simulink model "three_phase_pwm_rectifier_ac_dc_conv_simscape"  (R2019a)
settings: Solver=ode23t  StartTime=0.0  StopTime=2  MaxStep=1e-6  RelTol=1e-6
values from neighbouring files (symbols this model uses):
  Co = 10e-3    (= 0.01)    [design_parameters.m]
  fline = 50    [design_parameters.m]
  K = (3/2)*(Vm/Vdc)    (= 0.609375)    [design_parameters.m]
  Kic = Kpc/Tc    (= 4545.45454545)    [design_parameters.m]
  Kipll = Kpll/Tpll    [design_parameters.m]
  Kiv = Kpv/Tv    [design_parameters.m]
  Kpc = Kc    (= 90.9090909091)    [design_parameters.m]
  Kpll = (1/Vm)*(1/(alfa_pll*Tsamp))    [design_parameters.m]
  Kpv = Kv    [design_parameters.m]
  Ls = 10e-3    (= 0.01)    [design_parameters.m]
  Rload = 200    [design_parameters.m]
  Rs = 0.5    [design_parameters.m]
  T1 = Tsamp/10    (= 5e-06)    [design_parameters.m]
  T2 = Tsamp/10    (= 5e-06)    [design_parameters.m]
  Tsamp = Tsw/2    (= 5e-05)    [design_parameters.m]
  Vdc = 800    [design_parameters.m]
  Vm = 325    [design_parameters.m]
undefined symbols (not defined in the file or in its folder): Iqe_max
libraries: powerlib x32, simulink x4, powerlib_meascontrol x1
settings Model: Creator=Görkem  LastModifiedBy=gsahi
settings DataIOCC: ReturnWorkspaceOutputs=off
settings DebuggingCC: ParameterOverflowMsg=none

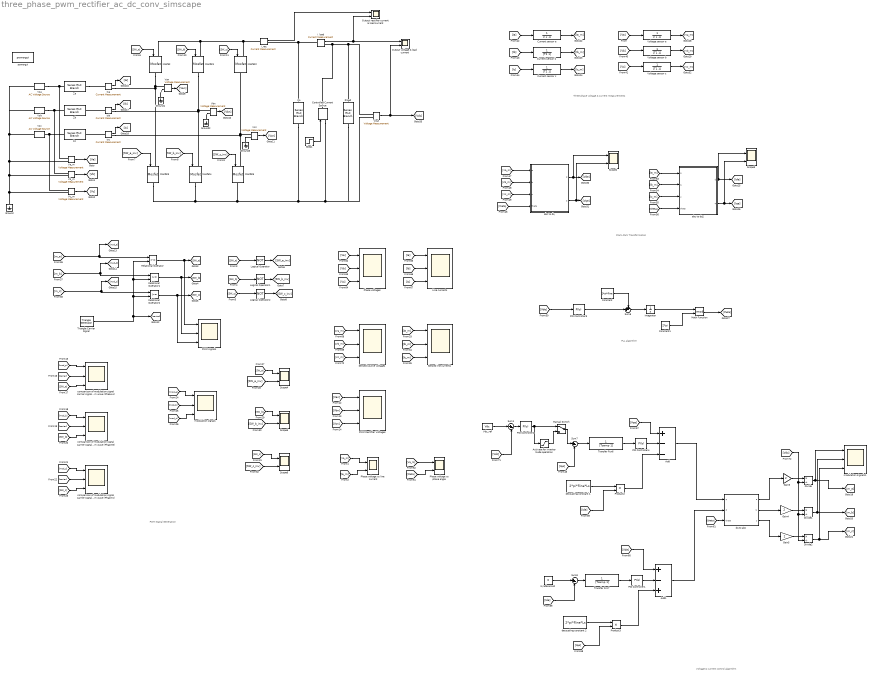
== system three_phase_pwm_rectifier_ac_dc_conv_simscape ==
  note: PWM Signal Generation
  note: Three phase voltage & current measurements
  note: Clark-Park Transformation
  note: PLL algorithm
  note: Voltage & current control algorithm
  "Activate for inverter mode operation " : Saturate  UpperLimit=-(Vdc/Rload)/K  LowerLimit=-20
  Add : Sum  Inputs=+--
  Add1 : Sum  Inputs=+-+
  Co : powerlib/Elements/Series RLC Branch  LConnTagsString=__new0  RConnTagsString=__new0  BranchType=C  Resistance=5  Inductance=1e-3  SetiL0=off  InitialCurrent=0  Capacitance=Co  Setx0=on  InitialVoltage=Vdc  Measurements=None
      settings: SourceProductName=Simscape Electrical
  Constant : Constant  Value=2*pi*fline
  Constant1 : Constant  Value=2*pi
  Controlled Current Source : powerlib/Electrical Sources/Controlled Current Source  Initialize=on  Source_Type=AC  Amplitude=0  Phase=0  Frequency=0  Measurements=None
      settings: SourceProductName=Simscape Electrical
  Current sensor a : TransferFcn  Denominator=[T2 1]
  Current sensor b : TransferFcn  Denominator=[T2 1]
  Current sensor c : TransferFcn  Denominator=[T2 1]
  Divide : Product  Inputs=*/
  Divide1 : Product  Inputs=*/
  Divide2 : Product  Inputs=*/
  Gain3 : Gain  Gain=2
  Gain4 : Gain  Gain=2
  Gain5 : Gain  Gain=2
  Ground{,1..3} (4 alike) : powerlib/Elements/Ground  LConnTagsString=a
      settings: SourceProductName=Simscape Electrical
  I_rec : powerlib/Measurements/Current Measurement  PhasorSimulation=off  OutputType=Complex  PSBequivalent=0
      settings: SourceProductName=Simscape Electrical
  Integrator : Integrator
  Iq reference2 : Constant  Value=0
  Isa : powerlib/Measurements/Current Measurement  PhasorSimulation=off  OutputType=Complex  PSBequivalent=0
      settings: SourceProductName=Simscape Electrical
  Isb : powerlib/Measurements/Current Measurement  PhasorSimulation=off  OutputType=Complex  PSBequivalent=0
      settings: SourceProductName=Simscape Electrical
  Isc : powerlib/Measurements/Current Measurement  PhasorSimulation=off  OutputType=Complex  PSBequivalent=0
      settings: SourceProductName=Simscape Electrical
  Line currents : Scope  NumInputPorts=3
  Logical Operator : Logic  Operator=NOT  AllPortsSameDT=off  OutDataTypeStr=boolean
  Logical Operator1 : Logic  Operator=NOT  AllPortsSameDT=off  OutDataTypeStr=boolean
  Logical Operator2 : Logic  Operator=NOT  AllPortsSameDT=off  OutDataTypeStr=boolean
  Manual Switch : ManualSwitch
  Math Function : Math  Operator=mod  SaturateOnIntegerOverflow=on
  Mosfet{,1..5} (6 alike) : powerlib/Power Electronics/Mosfet  Ron=0.1  Lon=0  Rd=0.01  Vfd=0  IC=0  Rs=1e5  Cs=inf  Measurements=off
      settings: SourceProductName=Simscape Electrical
  Output rectifier current & load current : Scope  NumInputPorts=2
  Output voltage & load current : Scope  NumInputPorts=2
  PID Controller1 : simulink/Continuous/PID Controller  Controller=PI  Form=Parallel  TimeDomain=Continuous-time  SampleTime=-1  IntegratorMethod=Forward Euler  FilterMethod=Forward Euler  ControllerParametersSource=internal  P=Kpc  I=Kic  D=0  UseFilter=on  N=100  TunerSelectOption=Transfer Function Based (PID Tuner App)  InitialConditionSource=internal  InitialConditionForIntegrator=0  InitialConditionForFilter=0  DifferentiatorICPrevScaledInput=0  ExternalReset=none  TrackingMode=off  Kt=1  LimitOutput=on  UpperSaturationLimit=400  LowerSaturationLimit=-400  LinearizeAsGain=on  AntiWindupMode=clamping  Kb=1  POutMin=[]  POutMax=[]  IOutMin=[]  IOutMax=[]  DOutMin=[]  DOutMax=[]  NOutMin=[]  NOutMax=[]  SumOutMin=[]  SumOutMax=[]  SaturationOutMin=[]  SaturationOutMax=[]  PParamMin=[]  PParamMax=[]  IParamMin=[]  IParamMax=[]  DParamMin=[]  DParamMax=[]  NParamMin=[]  NParamMax=[]  KbParamMin=[]  KbParamMax=[]  KtParamMin=[]  KtParamMax=[]  KbOutMin=[]  KbOutMax=[]  KtOutMin=[]  KtOutMax=[]  IntegratorOutMin=[]  IntegratorOutMax=[]  FilterOutMin=[]  FilterOutMax=[]  SumI1OutMin=[]  SumI1OutMax=[]  SumI2OutMin=[]  SumI2OutMax=[]  SumI3OutMin=[]  SumI3OutMax=[]  SumI4OutMin=[]  SumI4OutMax=[]  SumDOutMin=[]  SumDOutMax=[]  DifferentiatorOutMin=[]  DifferentiatorOutMax=[]  FilterDiffOutCoefMin=[]  FilterDiffOutCoefMax=[]  ReciprocalOutMin=[]  ReciprocalOutMax=[]  SumDenOutMin=[]  SumDenOutMax=[]  SumNumOutMin=[]  SumNumOutMax=[]  DivideOutMin=[]  DivideOutMax=[]  IntegratorContinuousStateAttributes=''  IntegratorStateMustResolveToSignalObject=off  IntegratorRTWStateStorageClass=Auto  FilterContinuousStateAttributes=''  FilterStateMustResolveToSignalObject=off  FilterRTWStateStorageClass=Auto  ParallelPVariant=InternalParameters  IdealPVariant=Disabled  IVariant=InternalParameters  DVariant=Disabled  IntegratorVariant=Continuous  SatVariant=Enabled  AWVariant=ContClampingParallel  PCopyVariant=Disabled  TRVariant=Disabled  FdbkBlocksVariant=Forward  IdealPFdbkVariant=Disabled  SatFdbkVariant=Disabled  DerivativeFilterVariant=Disabled  NVariant=Disabled  NCopyVariant=Disabled_SignalSpec  FilterICVariant=Disabled  IntegratorICVariant=InternalICs  ExternalResetVariant=Disabled  TRSumVariant=Passthrough  SumFdbkVariant=Disabled  SumVariant=Sum_PI
  PID Controller2 : simulink/Continuous/PID Controller  Controller=PI  Form=Parallel  TimeDomain=Continuous-time  SampleTime=-1  IntegratorMethod=Forward Euler  FilterMethod=Forward Euler  ControllerParametersSource=internal  P=Kpv  I=Kiv  D=0  UseFilter=on  N=100  TunerSelectOption=Transfer Function Based (PID Tuner App)  InitialConditionSource=internal  InitialConditionForIntegrator=0  InitialConditionForFilter=0  DifferentiatorICPrevScaledInput=0  ExternalReset=none  TrackingMode=off  Kt=1  LimitOutput=off  UpperSaturationLimit=Iqe_max  LowerSaturationLimit=-Iqe_max  LinearizeAsGain=on  AntiWindupMode=clamping  Kb=1  POutMin=[]  POutMax=[]  IOutMin=[]  IOutMax=[]  DOutMin=[]  DOutMax=[]  NOutMin=[]  NOutMax=[]  SumOutMin=[]  SumOutMax=[]  SaturationOutMin=[]  SaturationOutMax=[]  PParamMin=[]  PParamMax=[]  IParamMin=[]  IParamMax=[]  DParamMin=[]  DParamMax=[]  NParamMin=[]  NParamMax=[]  KbParamMin=[]  KbParamMax=[]  KtParamMin=[]  KtParamMax=[]  KbOutMin=[]  KbOutMax=[]  KtOutMin=[]  KtOutMax=[]  IntegratorOutMin=[]  IntegratorOutMax=[]  FilterOutMin=[]  FilterOutMax=[]  SumI1OutMin=[]  SumI1OutMax=[]  SumI2OutMin=[]  SumI2OutMax=[]  SumI3OutMin=[]  SumI3OutMax=[]  SumI4OutMin=[]  SumI4OutMax=[]  SumDOutMin=[]  SumDOutMax=[]  DifferentiatorOutMin=[]  DifferentiatorOutMax=[]  FilterDiffOutCoefMin=[]  FilterDiffOutCoefMax=[]  ReciprocalOutMin=[]  ReciprocalOutMax=[]  SumDenOutMin=[]  SumDenOutMax=[]  SumNumOutMin=[]  SumNumOutMax=[]  DivideOutMin=[]  DivideOutMax=[]  IntegratorContinuousStateAttributes=''  IntegratorStateMustResolveToSignalObject=off  IntegratorRTWStateStorageClass=Auto  FilterContinuousStateAttributes=''  FilterStateMustResolveToSignalObject=off  FilterRTWStateStorageClass=Auto  ParallelPVariant=InternalParameters  IdealPVariant=Disabled  IVariant=InternalParameters  DVariant=Disabled  IntegratorVariant=Continuous  SatVariant=Disabled  AWVariant=Passthrough  PCopyVariant=Disabled  TRVariant=Disabled  FdbkBlocksVariant=Forward  IdealPFdbkVariant=Disabled  SatFdbkVariant=Disabled  DerivativeFilterVariant=Disabled  NVariant=Disabled  NCopyVariant=Disabled_SignalSpec  FilterICVariant=Disabled  IntegratorICVariant=InternalICs  ExternalResetVariant=Disabled  TRSumVariant=Passthrough  SumFdbkVariant=Disabled  SumVariant=Sum_PI
  PID Controller3 : simulink/Continuous/PID Controller  Controller=PI  Form=Parallel  TimeDomain=Continuous-time  SampleTime=-1  IntegratorMethod=Forward Euler  FilterMethod=Forward Euler  ControllerParametersSource=internal  P=Kpll  I=Kipll  D=0  UseFilter=on  N=100  TunerSelectOption=Transfer Function Based (PID Tuner App)  InitialConditionSource=internal  InitialConditionForIntegrator=0  InitialConditionForFilter=0  DifferentiatorICPrevScaledInput=0  ExternalReset=none  TrackingMode=off  Kt=1  LimitOutput=off  UpperSaturationLimit=inf  LowerSaturationLimit=-inf  LinearizeAsGain=on  AntiWindupMode=none  Kb=1  POutMin=[]  POutMax=[]  IOutMin=[]  IOutMax=[]  DOutMin=[]  DOutMax=[]  NOutMin=[]  NOutMax=[]  SumOutMin=[]  SumOutMax=[]  SaturationOutMin=[]  SaturationOutMax=[]  PParamMin=[]  PParamMax=[]  IParamMin=[]  IParamMax=[]  DParamMin=[]  DParamMax=[]  NParamMin=[]  NParamMax=[]  KbParamMin=[]  KbParamMax=[]  KtParamMin=[]  KtParamMax=[]  KbOutMin=[]  KbOutMax=[]  KtOutMin=[]  KtOutMax=[]  IntegratorOutMin=[]  IntegratorOutMax=[]  FilterOutMin=[]  FilterOutMax=[]  SumI1OutMin=[]  SumI1OutMax=[]  SumI2OutMin=[]  SumI2OutMax=[]  SumI3OutMin=[]  SumI3OutMax=[]  SumI4OutMin=[]  SumI4OutMax=[]  SumDOutMin=[]  SumDOutMax=[]  DifferentiatorOutMin=[]  DifferentiatorOutMax=[]  FilterDiffOutCoefMin=[]  FilterDiffOutCoefMax=[]  ReciprocalOutMin=[]  ReciprocalOutMax=[]  SumDenOutMin=[]  SumDenOutMax=[]  SumNumOutMin=[]  SumNumOutMax=[]  DivideOutMin=[]  DivideOutMax=[]  IntegratorContinuousStateAttributes=''  IntegratorStateMustResolveToSignalObject=off  IntegratorRTWStateStorageClass=Auto  FilterContinuousStateAttributes=''  FilterStateMustResolveToSignalObject=off  FilterRTWStateStorageClass=Auto  ParallelPVariant=InternalParameters  IdealPVariant=Disabled  IVariant=InternalParameters  DVariant=Disabled  IntegratorVariant=Continuous  SatVariant=Disabled  AWVariant=Passthrough  PCopyVariant=Disabled  TRVariant=Disabled  FdbkBlocksVariant=Forward  IdealPFdbkVariant=Disabled  SatFdbkVariant=Disabled  DerivativeFilterVariant=Disabled  NVariant=Disabled  NCopyVariant=Disabled_SignalSpec  FilterICVariant=Disabled  IntegratorICVariant=InternalICs  ExternalResetVariant=Disabled  TRSumVariant=Passthrough  SumFdbkVariant=Disabled  SumVariant=Sum_PI
  PID Controller4 : simulink/Continuous/PID Controller  Controller=PI  Form=Parallel  TimeDomain=Continuous-time  SampleTime=-1  IntegratorMethod=Forward Euler  FilterMethod=Forward Euler  ControllerParametersSource=internal  P=Kpc  I=Kic  D=0  UseFilter=on  N=100  TunerSelectOption=Transfer Function Based (PID Tuner App)  InitialConditionSource=internal  InitialConditionForIntegrator=0  InitialConditionForFilter=0  DifferentiatorICPrevScaledInput=0  ExternalReset=none  TrackingMode=off  Kt=1  LimitOutput=on  UpperSaturationLimit=Vdc/2  LowerSaturationLimit=-Vdc/2  LinearizeAsGain=on  AntiWindupMode=clamping  Kb=1  POutMin=[]  POutMax=[]  IOutMin=[]  IOutMax=[]  DOutMin=[]  DOutMax=[]  NOutMin=[]  NOutMax=[]  SumOutMin=[]  SumOutMax=[]  SaturationOutMin=[]  SaturationOutMax=[]  PParamMin=[]  PParamMax=[]  IParamMin=[]  IParamMax=[]  DParamMin=[]  DParamMax=[]  NParamMin=[]  NParamMax=[]  KbParamMin=[]  KbParamMax=[]  KtParamMin=[]  KtParamMax=[]  KbOutMin=[]  KbOutMax=[]  KtOutMin=[]  KtOutMax=[]  IntegratorOutMin=[]  IntegratorOutMax=[]  FilterOutMin=[]  FilterOutMax=[]  SumI1OutMin=[]  SumI1OutMax=[]  SumI2OutMin=[]  SumI2OutMax=[]  SumI3OutMin=[]  SumI3OutMax=[]  SumI4OutMin=[]  SumI4OutMax=[]  SumDOutMin=[]  SumDOutMax=[]  DifferentiatorOutMin=[]  DifferentiatorOutMax=[]  FilterDiffOutCoefMin=[]  FilterDiffOutCoefMax=[]  ReciprocalOutMin=[]  ReciprocalOutMax=[]  SumDenOutMin=[]  SumDenOutMax=[]  SumNumOutMin=[]  SumNumOutMax=[]  DivideOutMin=[]  DivideOutMax=[]  IntegratorContinuousStateAttributes=''  IntegratorStateMustResolveToSignalObject=off  IntegratorRTWStateStorageClass=Auto  FilterContinuousStateAttributes=''  FilterStateMustResolveToSignalObject=off  FilterRTWStateStorageClass=Auto  ParallelPVariant=InternalParameters  IdealPVariant=Disabled  IVariant=InternalParameters  DVariant=Disabled  IntegratorVariant=Continuous  SatVariant=Enabled  AWVariant=ContClampingParallel  PCopyVariant=Disabled  TRVariant=Disabled  FdbkBlocksVariant=Forward  IdealPFdbkVariant=Disabled  SatFdbkVariant=Disabled  DerivativeFilterVariant=Disabled  NVariant=Disabled  NCopyVariant=Disabled_SignalSpec  FilterICVariant=Disabled  IntegratorICVariant=InternalICs  ExternalResetVariant=Disabled  TRSumVariant=Passthrough  SumFdbkVariant=Disabled  SumVariant=Sum_PI
  PWM Rectifier Voltages : Scope  NumInputPorts=3
  PWM signals : Scope  NumInputPorts=3
  Phase voltage vs line current : Scope  NumInputPorts=2
  Phase voltage vs phase angle : Scope  NumInputPorts=2
  Phase voltages : Scope  NumInputPorts=3
  Product2 : Product
  Product3 : Product
  Relational Operator : RelationalOperator  OutDataTypeStr=boolean  RndMeth=Simplest
  Relational Operator1 : RelationalOperator  OutDataTypeStr=boolean  RndMeth=Simplest
  Relational Operator2 : RelationalOperator  OutDataTypeStr=boolean  RndMeth=Simplest
  Rload : powerlib/Elements/Series RLC Branch  LConnTagsString=__new0  RConnTagsString=__new0  BranchType=R  Resistance=Rload  Inductance=1e-3  SetiL0=off  InitialCurrent=0  Capacitance=Co  Setx0=on  InitialVoltage=Vdc  Measurements=None
      settings: SourceProductName=Simscape Electrical
  Scope{2..6} (5 alike) : Scope  NumInputPorts=2
  Sensed line currents : Scope  NumInputPorts=3
  Sensed source voltages : Scope  NumInputPorts=3
  Step1 : Step  Time=0.05  After=-Vdc/(3*Rload)  SampleTime=0
  Sum1 : Sum  Inputs=|+-
  Sum6 : Sum  Inputs=++|
  Sum7 : Sum  Inputs=|+-
  Sum8 : Sum  Inputs=|+-
  Transfer Fcn6 : TransferFcn  Denominator=[Tsamp 1]
  Transfer Fcn7 : TransferFcn  Denominator=[Tsamp 1]
  Triangle Carrier Signal : powerlib_meascontrol/Pulse & Signal Generators/Triangle Generator  Freq=fsw  Phase=-90  Ts=0
      settings: SourceProductName=Simscape Electrical
  Va_m : powerlib/Measurements/Voltage Measurement  PhasorSimulation=off  OutputType=Complex  PSBequivalent=0
      settings: SourceProductName=Simscape Electrical
  Van : powerlib/Measurements/Voltage Measurement  PhasorSimulation=off  OutputType=Complex  PSBequivalent=0
      settings: SourceProductName=Simscape Electrical
  Vb_m : powerlib/Measurements/Voltage Measurement  PhasorSimulation=off  OutputType=Complex  PSBequivalent=0
      settings: SourceProductName=Simscape Electrical
  Vbn : powerlib/Measurements/Voltage Measurement  PhasorSimulation=off  OutputType=Complex  PSBequivalent=0
      settings: SourceProductName=Simscape Electrical
  Vc_m : powerlib/Measurements/Voltage Measurement  PhasorSimulation=off  OutputType=Complex  PSBequivalent=0
      settings: SourceProductName=Simscape Electrical
  Vcn : powerlib/Measurements/Voltage Measurement  PhasorSimulation=off  OutputType=Complex  PSBequivalent=0
      settings: SourceProductName=Simscape Electrical
  Vdc_ref : Constant  Value=Vdc
  Voltage sensor a : TransferFcn  Denominator=[T1 1]
  Voltage sensor b : TransferFcn  Denominator=[T1 1]
  Voltage sensor c : TransferFcn  Denominator=[T1 1]
  Vout : powerlib/Measurements/Voltage Measurement  PhasorSimulation=off  OutputType=Complex  PSBequivalent=0
      settings: SourceProductName=Simscape Electrical
  Vsa : powerlib/Electrical Sources/AC Voltage Source  Amplitude=Vm  Phase=0  Frequency=fline  SampleTime=0  Measurements=None  BusType=swing  Pref=10e3  Qref=0  Qmin=-inf  Qmax=+inf
      settings: SourceProductName=Simscape Electrical
  Vsb : powerlib/Electrical Sources/AC Voltage Source  Amplitude=Vm  Phase=-120  Frequency=fline  SampleTime=0  Measurements=None  BusType=swing  Pref=10e3  Qref=0  Qmin=-inf  Qmax=+inf
      settings: SourceProductName=Simscape Electrical
  Vsc : powerlib/Electrical Sources/AC Voltage Source  Amplitude=Vm  Phase=-240  Frequency=fline  SampleTime=0  Measurements=None  BusType=swing  Pref=10e3  Qref=0  Qmin=-inf  Qmax=+inf
      settings: SourceProductName=Simscape Electrical
  Za : powerlib/Elements/Series RLC Branch  LConnTagsString=__new0  RConnTagsString=__new0  BranchType=RL  Resistance=Rs  Inductance=Ls  SetiL0=off  InitialCurrent=0  Capacitance=1e-6  Setx0=off  InitialVoltage=0  Measurements=None
      settings: SourceProductName=Simscape Electrical
  Zb : powerlib/Elements/Series RLC Branch  LConnTagsString=__new0  RConnTagsString=__new0  BranchType=RL  Resistance=Rs  Inductance=Ls  SetiL0=off  InitialCurrent=0  Capacitance=1e-6  Setx0=off  InitialVoltage=0  Measurements=None
      settings: SourceProductName=Simscape Electrical
  Zc : powerlib/Elements/Series RLC Branch  LConnTagsString=__new0  RConnTagsString=__new0  BranchType=RL  Resistance=Rs  Inductance=Ls  SetiL0=off  InitialCurrent=0  Capacitance=1e-6  Setx0=off  InitialVoltage=0  Measurements=None
      settings: SourceProductName=Simscape Electrical
  abc to dq : Subsystem
  abc to dq2 : Subsystem
  comparison of modulation signal carrier signal and pwm wave (Phase A) : Scope  NumInputPorts=3
  comparison of modulation signal carrier signal and pwm wave (Phase B) : Scope  NumInputPorts=3
  comparison of modulation signal carrier signal and pwm wave (Phase C) : Scope  NumInputPorts=3
  decoupling constant 1 : Constant  Value=2*pi*fline*Ls
  decoupling constant 2 : Constant  Value=2*pi*fline*Ls
  dq to abc : Subsystem
  i_load : powerlib/Measurements/Current Measurement  PhasorSimulation=off  OutputType=Complex  PSBequivalent=0
      settings: SourceProductName=Simscape Electrical
  modulation signals : Scope  NumInputPorts=3
  modulation signals1 : Scope  NumInputPorts=3
  powergui : powerlib/powergui  Priority=1  SimulationMode=Continuous  SampleTime=50e-6  frequency=60  Iterations=50  frequencyindice=50  Pbase=100e6  ErrMax=1e-4  UnitsV=kV  UnitsW=MW  buscounter=0  FunctionMessages=off  echomessages=off  EnableUseOfTLC=off  CurrentSourceSwitches=off  DisableSnubberDevices=off  DisableRonSwitches=off  DisableVfSwitches=off  DisplayEquations=off  AutomaticDiscreteSolvers=off  SolverType=Tustin/Backward Euler (TBE)  Interpol=off  ExternalGateDelay=off  methode=off  Ts=100  x0status=blocks  SPID=on  SwTol=0  HookPort=off  NonlinearTolerance=0  nMaxIteration=15  ContinueOnMaxIteration=off  RestoreLinks=warning  ResistiveCurrentMeasurement=off  Frange=[0:2:500]  Ylog=off  Xlog=on  ShowGrid=off  save=off  variable=ZData  structure=0  ZoomFFT=off  StartTime=0.0  cycles=1  DisplayStyle=1  fundamental=60  FreqAxis=off  MaxFrequency=1000  frequencyindicesteady=1  RmsSteady=1  display=off
      settings: SourceProductName=Simscape Electrical
  wires:
  Va_m/1 -> [Va]
  Vb_m/1 -> [Vb]
  Vc_m/1 -> [Vc]
  Triangle Carrier Signal/1 -> [carrier], Relational Operator2/2, Relational Operator1/2, Relational Operator/2
  [m_b] -> Relational Operator1/1, [mod_b]
  [m_c] -> Relational Operator2/1, [mod_c]
  Relational Operator/1 -> PWM signals/1, [SW_a]
  Relational Operator1/1 -> PWM signals/2, [SW_b]
  Relational Operator2/1 -> PWM signals/3, [SW_c]
  [SW_a] -> Logical Operator/1
  [SW_c] -> Logical Operator2/1
  [SW_b] -> Logical Operator1/1
  Logical Operator/1 -> [SW_a_inv]
  Logical Operator1/1 -> [SW_b_inv]
  Logical Operator2/1 -> [SW_c_inv]
  [SW_a] -> Mosfet/1
  [SW_a_inv] -> Mosfet3/1
  [SW_b_inv] -> Mosfet4/1
  [SW_c_inv] -> Mosfet5/1
  Vout/1 -> [Vdc], Output voltage & load current/2
  i_load/1 -> Output rectifier current & load current/2, Output voltage & load current/1
  I_rec/1 -> Output rectifier current & load current/1
  [SW_b] -> Mosfet1/1
  [SW_c] -> Mosfet2/1
  Van/1 -> [Van]
  Vbn/1 -> [Vbn]
  Vcn/1 -> [Vcn]
  [Van] -> PWM Rectifier Voltages/1
  [Vbn] -> PWM Rectifier Voltages/2
  [Vcn] -> PWM Rectifier Voltages/3
  [m_a] -> Relational Operator/1, [mod_a]
  [mod_a] -> comparison of modulation signal carrier signal and pwm wave (Phase A)/1
  [carrier] -> comparison of modulation signal carrier signal and pwm wave (Phase A)/2
  [SW_a] -> comparison of modulation signal carrier signal and pwm wave (Phase A)/3
  [SW_b] -> comparison of modulation signal carrier signal and pwm wave (Phase B)/3
  [mod_b] -> comparison of modulation signal carrier signal and pwm wave (Phase B)/1
  [carrier] -> comparison of modulation signal carrier signal and pwm wave (Phase B)/2
  [SW_c] -> comparison of modulation signal carrier signal and pwm wave (Phase C)/3
  [mod_c] -> comparison of modulation signal carrier signal and pwm wave (Phase C)/1
  [carrier] -> comparison of modulation signal carrier signal and pwm wave (Phase C)/2
  [mod_b] -> modulation signals/2
  [mod_a] -> modulation signals/1
  [mod_c] -> modulation signals/3
  [SW_a] -> Scope4/1
  [SW_a_inv] -> Scope4/2
  [SW_b] -> Scope5/1
  [SW_b_inv] -> Scope5/2
  [SW_c_inv] -> Scope6/2
  [SW_c] -> Scope6/1
  Isa/1 -> [Ia]
  Isb/1 -> [Ib]
  Isc/1 -> [Ic]
  [Ia_m] -> Sensed line currents/1
  [Ib_m] -> Sensed line currents/2
  [Ic_m] -> Sensed line currents/3
  abc to dq/2(q) -> Scope2/2, [Vqe]
  abc to dq/1(d) -> Scope2/1, [Vde]
  [theta] -> abc to dq/4(theta)
  [Va_m] -> abc to dq/1(a)
  [Vb_m] -> abc to dq/2(b)
  [Vc_m] -> abc to dq/3(c)
  [Va_m] -> Phase voltage vs phase angle/1
  [theta] -> Phase voltage vs phase angle/2
  [Ia_m] -> abc to dq2/1(a)
  [Ib_m] -> abc to dq2/2(b)
  [Ic_m] -> abc to dq2/3(c)
  [theta] -> abc to dq2/4(theta)
  abc to dq2/1(d) -> Scope3/1, [Ide]
  abc to dq2/2(q) -> Scope3/2, [Iqe]
  [Ia_m] -> Phase voltage vs line current/2
  [Va_m] -> Phase voltage vs line current/1
  [Ia] -> Current sensor a/1
  [Ib] -> Current sensor b/1
  [Ic] -> Current sensor c/1
  Current sensor a/1 -> [Ia_m]
  Current sensor b/1 -> [Ib_m]
  Current sensor c/1 -> [Ic_m]
  [Vc] -> Voltage sensor c/1
  [Vb] -> Voltage sensor b/1
  [Va] -> Voltage sensor a/1
  Voltage sensor a/1 -> [Va_m]
  Voltage sensor b/1 -> [Vb_m]
  Voltage sensor c/1 -> [Vc_m]
  Product2/1 -> Add/3
  Add/1 -> dq to abc/1(q)
  PID Controller1/1 -> Add1/2
  decoupling constant 1/1 -> Product2/1
  Transfer Fcn7/1 -> PID Controller1/1
  Transfer Fcn6/1 -> PID Controller4/1
  decoupling constant 2/1 -> Product3/1
  Sum8/1 -> Transfer Fcn7/1
  [theta] -> dq to abc/3(theta)
  PID Controller4/1 -> Add/2
  Math Function/1 -> [theta]
  Sum6/1 -> Integrator/1
  Constant1/1 -> Math Function/2
  Add1/1 -> dq to abc/2(d)
  Sum7/1 -> Transfer Fcn6/1
  Constant/1 -> Sum6/1
  Product3/1 -> Add1/3
  PID Controller3/1 -> Sum6/2
  Integrator/1 -> Math Function/1
  [Vde] -> PID Controller3/1
  [Vqe] -> Add/1
  Iq reference2/1 -> Sum8/1
  [Ide] -> Sum8/2
  [Ide] -> Product2/2
  [Iqe] -> Product3/2
  [Vde] -> Add1/1
  [Va] -> Phase voltages/1
  [Vb] -> Phase voltages/2
  [Vc] -> Phase voltages/3
  [Ia] -> Line currents/1
  [Ib] -> Line currents/2
  [Ic] -> Line currents/3
  [Va_m] -> Sensed source voltages/1
  [Vb_m] -> Sensed source voltages/2
  [Vc_m] -> Sensed source voltages/3
  Sum1/1 -> PID Controller2/1
  [Iqe] -> Sum7/2
  "Activate for inverter mode operation "/1 -> Manual Switch/2
  dq to abc/1(a) -> Gain3/1
  dq to abc/2(b) -> Gain4/1
  dq to abc/3(c) -> Gain5/1
  Gain3/1 -> Divide/1
  Gain4/1 -> Divide1/1
  Gain5/1 -> Divide2/1
  [Vdc] -> Divide2/2, Divide1/2, Divide/2
  Divide1/1 -> modulation signals1/2, [m_b]
  Divide2/1 -> modulation signals1/3, [m_c]
  Divide/1 -> modulation signals1/1, [m_a]
  PID Controller2/1 -> Manual Switch/1, "Activate for inverter mode operation "/1
  Step1/1 -> Controlled Current Source/1
  Manual Switch/1 -> Sum7/1
  Vdc_ref/1 -> Sum1/1
  [Vdc] -> Sum1/2
  connections:
  Ground/LConn1 -- Vb_m/LConn2 -- Vsb/LConn1 -- Vsa/LConn1 -- Vsc/LConn1 -- Va_m/LConn2 -- Vc_m/LConn2
  Vsa/RConn1 -- Va_m/LConn1 -- Za/LConn1
  Vsb/RConn1 -- Vb_m/LConn1 -- Zb/LConn1
  Vsc/RConn1 -- Vc_m/LConn1 -- Zc/LConn1
  Mosfet5/LConn1 -- Vcn/LConn1 -- Mosfet2/RConn1 -- Isc/RConn1
  Mosfet1/RConn1 -- Isb/RConn1 -- Mosfet4/LConn1 -- Vbn/LConn1
  Mosfet/RConn1 -- Mosfet3/LConn1 -- Isa/RConn1 -- Van/LConn1
  Mosfet3/RConn1 -- Mosfet4/RConn1 -- Controlled Current Source/LConn1 -- Vout/LConn2 -- Rload/RConn1 -- Co/RConn1 -- Mosfet5/RConn1
  Mosfet/LConn1 -- Mosfet1/LConn1 -- I_rec/LConn1 -- Mosfet2/LConn1
  i_load/LConn1 -- I_rec/RConn1 -- Co/LConn1
  Vout/LConn1 -- Rload/LConn1 -- Controlled Current Source/RConn1 -- i_load/RConn1
  Ground1/LConn1 -- Van/LConn2
  Ground2/LConn1 -- Vbn/LConn2
  Ground3/LConn1 -- Vcn/LConn2
  Za/RConn1 -- Isa/LConn1
  Isb/LConn1 -- Zb/RConn1
  Isc/LConn1 -- Zc/RConn1

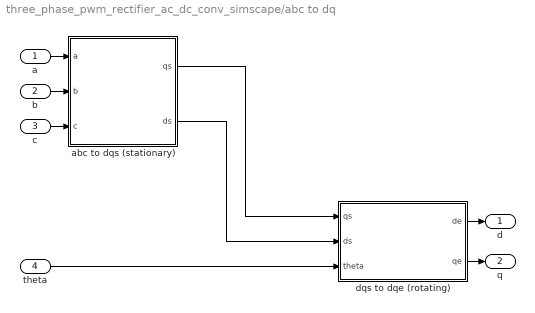
== system three_phase_pwm_rectifier_ac_dc_conv_simscape/abc to dq ==
  a : Inport
  b : Inport  Port=2
  c : Inport  Port=3
  theta : Inport  Port=4
  abc to dqs (stationary) : Subsystem
  dqs to dqe (rotating) : Subsystem
  d : Outport
  q : Outport  Port=2
  wires:
  abc to dqs (stationary)/1(qs) -> dqs to dqe (rotating)/1("qs ")
  dqs to dqe (rotating)/2("qe ") -> q/1
  abc to dqs (stationary)/2(ds) -> dqs to dqe (rotating)/2("ds ")
  a/1 -> abc to dqs (stationary)/1(a)
  b/1 -> abc to dqs (stationary)/2(b)
  c/1 -> abc to dqs (stationary)/3(c)
  dqs to dqe (rotating)/1("de ") -> d/1
  theta/1 -> dqs to dqe (rotating)/3(theta)

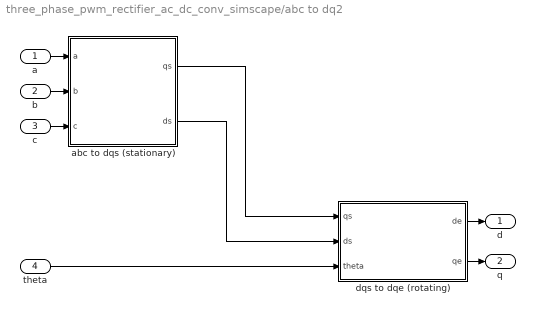
== system three_phase_pwm_rectifier_ac_dc_conv_simscape/abc to dq2 ==
  a : Inport
  b : Inport  Port=2
  c : Inport  Port=3
  theta : Inport  Port=4
  abc to dqs (stationary) : Subsystem
  dqs to dqe (rotating) : Subsystem
  d : Outport
  q : Outport  Port=2
  wires:
  abc to dqs (stationary)/1(qs) -> dqs to dqe (rotating)/1("qs ")
  dqs to dqe (rotating)/2("qe ") -> q/1
  abc to dqs (stationary)/2(ds) -> dqs to dqe (rotating)/2("ds ")
  a/1 -> abc to dqs (stationary)/1(a)
  b/1 -> abc to dqs (stationary)/2(b)
  c/1 -> abc to dqs (stationary)/3(c)
  dqs to dqe (rotating)/1("de ") -> d/1
  theta/1 -> dqs to dqe (rotating)/3(theta)

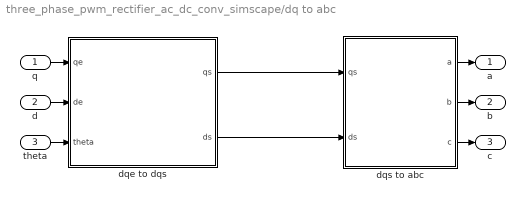
== system three_phase_pwm_rectifier_ac_dc_conv_simscape/dq to abc ==
  q : Inport
  d : Inport  Port=2
  theta : Inport  Port=3
  dqe to dqs : Subsystem
  dqs to abc : Subsystem
  a : Outport
  b : Outport  Port=2
  c : Outport  Port=3
  wires:
  d/1 -> dqe to dqs/2("de ")
  dqe to dqs/1("qs ") -> dqs to abc/1(qs)
  q/1 -> dqe to dqs/1("qe ")
  dqe to dqs/2(ds) -> dqs to abc/2(ds)
  dqs to abc/3(c) -> c/1
  dqs to abc/2(b) -> b/1
  dqs to abc/1(a) -> a/1
  theta/1 -> dqe to dqs/3(theta)

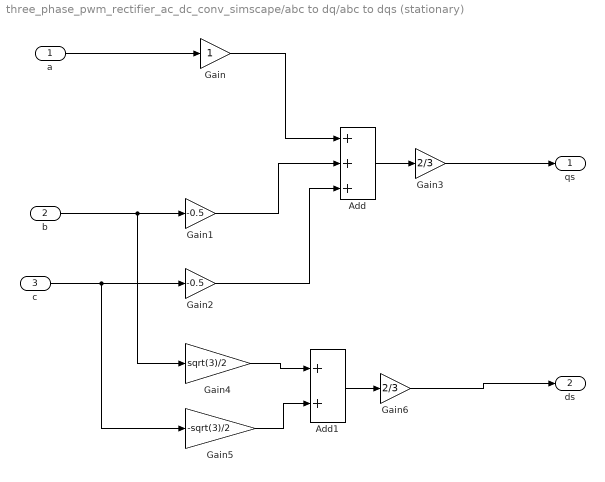
== system three_phase_pwm_rectifier_ac_dc_conv_simscape/abc to dq/abc to dqs (stationary) ==
  a : Inport
  b : Inport  Port=2
  c : Inport  Port=3
  Add : Sum  Inputs=+++
  Add1 : Sum
  Gain : Gain
  Gain1 : Gain  Gain=-0.5
  Gain2 : Gain  Gain=-0.5
  Gain3 : Gain  Gain=2/3
  Gain4 : Gain  Gain=sqrt(3)/2
  Gain5 : Gain  Gain=-sqrt(3)/2
  Gain6 : Gain  Gain=2/3
  qs : Outport
  ds : Outport  Port=2
  wires:
  a/1 -> Gain/1
  Gain/1 -> Add/1
  Gain5/1 -> Add1/2
  Gain1/1 -> Add/2
  b/1 -> Gain4/1, Gain1/1
  c/1 -> Gain5/1, Gain2/1
  Add/1 -> Gain3/1
  Gain2/1 -> Add/3
  Gain4/1 -> Add1/1
  Gain3/1 -> qs/1
  Add1/1 -> Gain6/1
  Gain6/1 -> ds/1

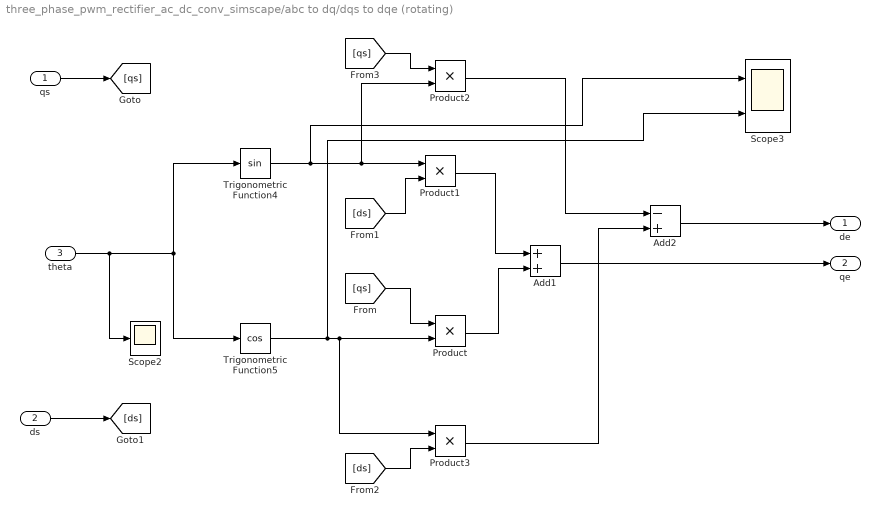
== system three_phase_pwm_rectifier_ac_dc_conv_simscape/abc to dq/dqs to dqe (rotating) ==
  "qs " : Inport
  "ds " : Inport  Port=2
  theta : Inport  Port=3
  Add1 : Sum
  Add2 : Sum  Inputs=-+
  Product{,1..3} (4 alike) : Product
  Scope2 : Scope
  Scope3 : Scope  NumInputPorts=2
  Trigonometric Function4 : Trigonometry
  Trigonometric Function5 : Trigonometry  Operator=cos
  "de " : Outport
  "qe " : Outport  Port=2
  wires:
  [ds] -> Product3/2
  theta/1 -> Scope2/1, Trigonometric Function4/1, Trigonometric Function5/1
  "ds "/1 -> [ds]
  Add2/1 -> "de "/1
  Product2/1 -> Add2/1
  [qs] -> Product/1
  "qs "/1 -> [qs]
  Product3/1 -> Add2/2
  [qs] -> Product2/1
  Add1/1 -> "qe "/1
  [ds] -> Product1/2
  Product/1 -> Add1/2
  Product1/1 -> Add1/1
  Trigonometric Function4/1 -> Product2/2, Product1/1, Scope3/1
  Trigonometric Function5/1 -> Product/2, Product3/1, Scope3/2

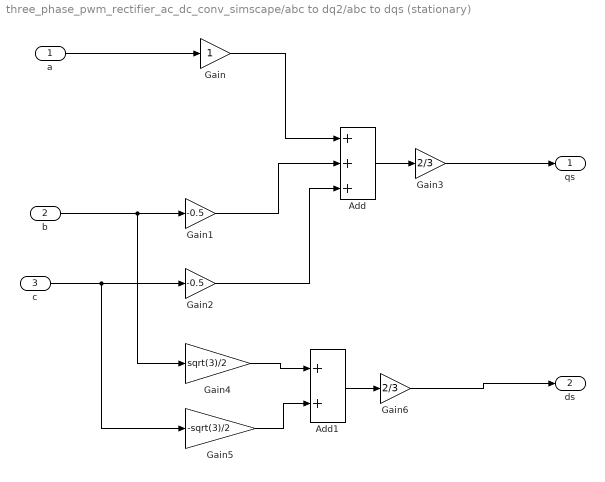
== system three_phase_pwm_rectifier_ac_dc_conv_simscape/abc to dq2/abc to dqs (stationary) ==
  a : Inport
  b : Inport  Port=2
  c : Inport  Port=3
  Add : Sum  Inputs=+++
  Add1 : Sum
  Gain : Gain
  Gain1 : Gain  Gain=-0.5
  Gain2 : Gain  Gain=-0.5
  Gain3 : Gain  Gain=2/3
  Gain4 : Gain  Gain=sqrt(3)/2
  Gain5 : Gain  Gain=-sqrt(3)/2
  Gain6 : Gain  Gain=2/3
  qs : Outport
  ds : Outport  Port=2
  wires:
  a/1 -> Gain/1
  Gain/1 -> Add/1
  Gain5/1 -> Add1/2
  Gain1/1 -> Add/2
  b/1 -> Gain4/1, Gain1/1
  c/1 -> Gain5/1, Gain2/1
  Add/1 -> Gain3/1
  Gain2/1 -> Add/3
  Gain4/1 -> Add1/1
  Gain3/1 -> qs/1
  Add1/1 -> Gain6/1
  Gain6/1 -> ds/1

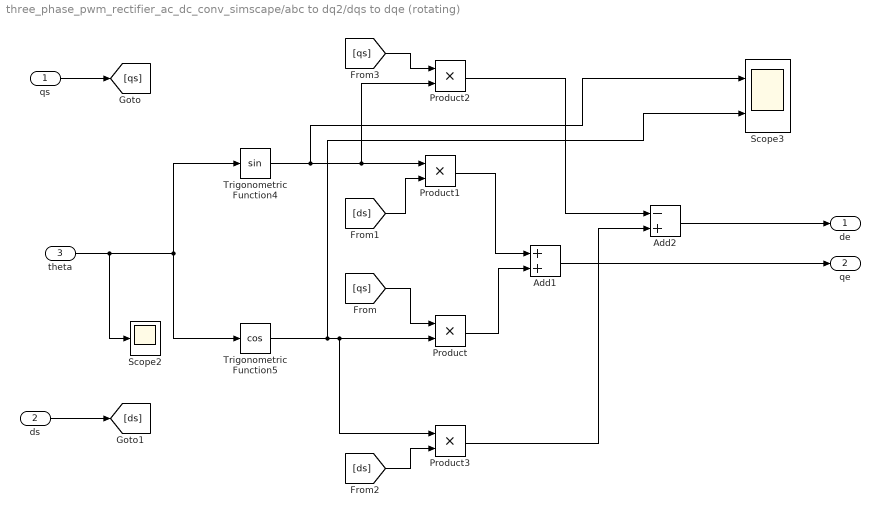
== system three_phase_pwm_rectifier_ac_dc_conv_simscape/abc to dq2/dqs to dqe (rotating) ==
  "qs " : Inport
  "ds " : Inport  Port=2
  theta : Inport  Port=3
  Add1 : Sum
  Add2 : Sum  Inputs=-+
  Product{,1..3} (4 alike) : Product
  Scope2 : Scope
  Scope3 : Scope  NumInputPorts=2
  Trigonometric Function4 : Trigonometry
  Trigonometric Function5 : Trigonometry  Operator=cos
  "de " : Outport
  "qe " : Outport  Port=2
  wires:
  [ds] -> Product3/2
  theta/1 -> Scope2/1, Trigonometric Function4/1, Trigonometric Function5/1
  "ds "/1 -> [ds]
  Add2/1 -> "de "/1
  Product2/1 -> Add2/1
  [qs] -> Product/1
  "qs "/1 -> [qs]
  Product3/1 -> Add2/2
  [qs] -> Product2/1
  Add1/1 -> "qe "/1
  [ds] -> Product1/2
  Product/1 -> Add1/2
  Product1/1 -> Add1/1
  Trigonometric Function4/1 -> Product2/2, Product1/1, Scope3/1
  Trigonometric Function5/1 -> Product/2, Product3/1, Scope3/2

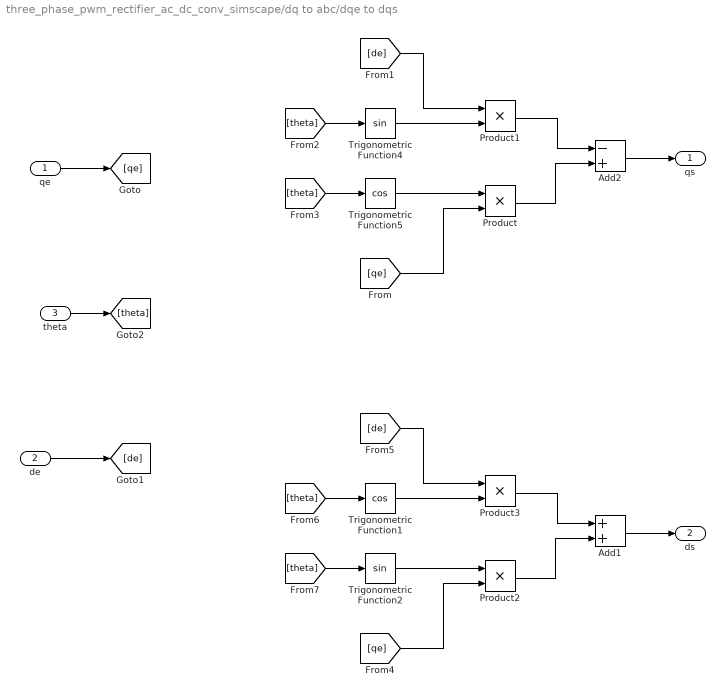
== system three_phase_pwm_rectifier_ac_dc_conv_simscape/dq to abc/dqe to dqs ==
  "qe " : Inport
  "de " : Inport  Port=2
  theta : Inport  Port=3
  Add1 : Sum
  Add2 : Sum  Inputs=-+
  Product{,1..3} (4 alike) : Product
  Trigonometric Function1 : Trigonometry  Operator=cos
  Trigonometric Function2 : Trigonometry
  Trigonometric Function4 : Trigonometry
  Trigonometric Function5 : Trigonometry  Operator=cos
  "qs " : Outport
  ds : Outport  Port=2
  wires:
  "de "/1 -> [de]
  Add2/1 -> "qs "/1
  "qe "/1 -> [qe]
  Trigonometric Function5/1 -> Product/1
  [qe] -> Product/2
  Trigonometric Function4/1 -> Product1/2
  [de] -> Product1/1
  Product1/1 -> Add2/1
  Product/1 -> Add2/2
  theta/1 -> [theta]
  [theta] -> Trigonometric Function4/1
  [theta] -> Trigonometric Function5/1
  Trigonometric Function1/1 -> Product3/2
  [theta] -> Trigonometric Function2/1
  [theta] -> Trigonometric Function1/1
  Product2/1 -> Add1/2
  [de] -> Product3/1
  [qe] -> Product2/2
  Trigonometric Function2/1 -> Product2/1
  Add1/1 -> ds/1
  Product3/1 -> Add1/1

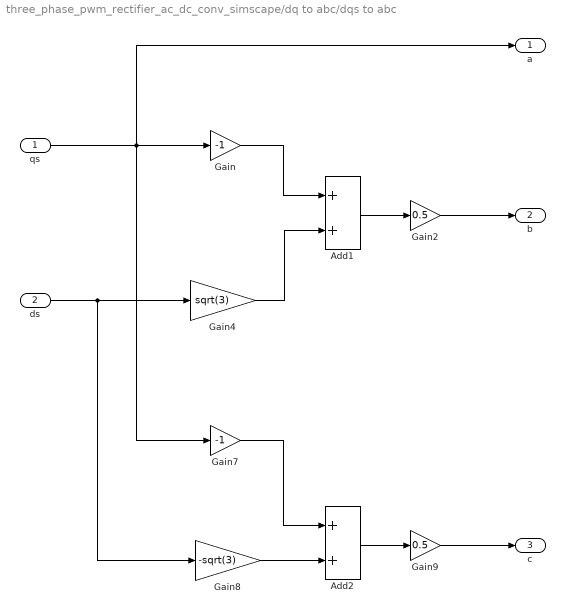
== system three_phase_pwm_rectifier_ac_dc_conv_simscape/dq to abc/dqs to abc ==
  qs : Inport
  ds : Inport  Port=2
  Add1 : Sum
  Add2 : Sum
  Gain : Gain  Gain=-1
  Gain2 : Gain  Gain=0.5
  Gain4 : Gain  Gain=sqrt(3)
  Gain7 : Gain  Gain=-1
  Gain8 : Gain  Gain=-sqrt(3)
  Gain9 : Gain  Gain=0.5
  a : Outport
  b : Outport  Port=2
  c : Outport  Port=3
  wires:
  qs/1 -> Gain7/1, a/1, Gain/1
  ds/1 -> Gain8/1, Gain4/1
  Gain/1 -> Add1/1
  Gain4/1 -> Add1/2
  Add1/1 -> Gain2/1
  Gain2/1 -> b/1
  Gain7/1 -> Add2/1
  Gain8/1 -> Add2/2
  Add2/1 -> Gain9/1
  Gain9/1 -> c/1
